simulink model "simu_unsteady_validation"  (R2020a)
settings: Solver=VariableStepAuto  StartTime=0.0  StopTime=t_final  RelTol=1e-3
values from neighbouring files (symbols this model uses):
  A_lti = - M \ L    [main_unsteady.m]    (also in main_unsteady_validation.m)
  B_lti = M \ [f_omega f_gammaR1 f_gammaQ]    [main_unsteady.m]    (also in main_unsteady_validation.m)
  C_lti = eye(size(A_lti))    [main_unsteady.m]    (also in main_unsteady_validation.m)
  D_lti = zeros(size(B_lti))    [main_unsteady.m]    (also in main_unsteady_validation.m)
  q0 = 0    [main_steadyState.m]    (also in main_steadyState_validation.m; main_unsteady.m; main_unsteady_validation.m)
  T = 20    [main_steadyState.m]    (also in main_steadyState_validation.m = 0; main_unsteady.m = 10; main_unsteady_validation.m = 0)
  THETA_0 = zeros(n_dof,1) + T    [main_unsteady.m]    (also in main_unsteady_validation.m = (exp(p(nodes_coordinates_full(1,:))) .* exp(g(nodes_coordina)
libraries: simulink x1
settings Model: Creator=luigidamico  LastModifiedBy=luigidamico

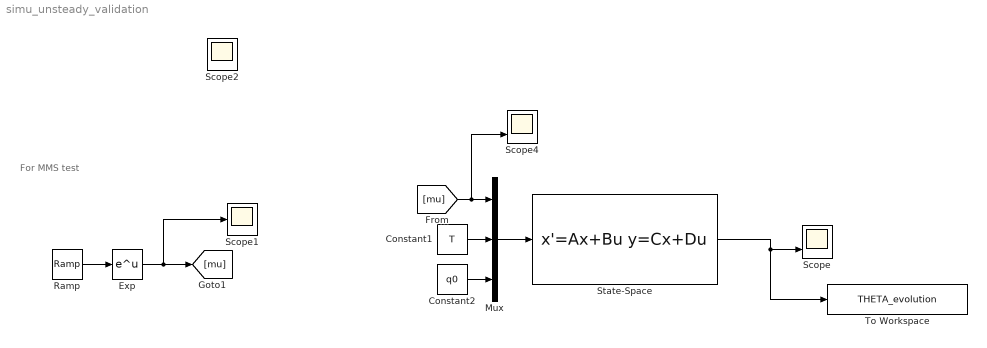
== system simu_unsteady_validation ==
  note: For MMS test
  Constant1 : Constant  Value=T
  Constant2 : Constant  Value=q0
  Exp : Math  SaturateOnIntegerOverflow=on
  Mux : Mux  Inputs=3
  Ramp : simulink/Sources/Ramp  slope=-1/20  start=0  InitialOutput=0
  Scope : Scope  NumInputPorts=2
  Scope1 : Scope
  Scope4 : Scope  NumInputPorts=2
  State-Space : StateSpace  A=A_lti  B=B_lti  C=C_lti  D=D_lti  InitialCondition=THETA_0
  To Workspace : ToWorkspace  VariableName=THETA_evolution  SaveFormat=Timeseries  SampleTime=-1
  Scope2 : Scope
  wires:
  Mux/1 -> State-Space/1
  Constant2/1 -> Mux/3
  State-Space/1 -> To Workspace/1, Scope/2
  Ramp/1 -> Exp/1
  Exp/1 -> Scope1/1, [mu]
  [mu] -> Scope4/2, Mux/1
  Constant1/1 -> Mux/2
